simulink model "test_scan"  (Simulink 6.5)
settings: Solver=VariableStepDiscrete  StartTime=0.0  StopTime=5000  RelTol=1e-3
undefined symbols (not defined in the file or in its folder): sigbuilder_block
libraries: xbsIndex_r4 x78, nort_sysgenlib x8
settings Model: Creator=nort  LastModifiedBy=nort

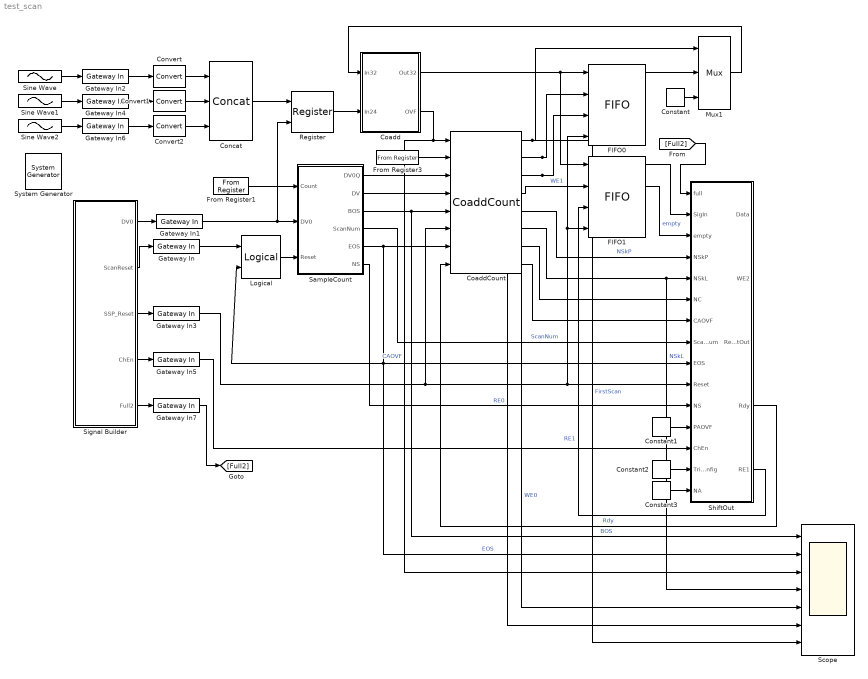
== system test_scan ==
  " System Generator" : xbsIndex_r4/ System Generator  Tag=genX  SystemSampleTime=-1  xilinxfamily=Virtex4  part=xc4vsx35  speed=-10  package=ff668  synthesis_tool=XST  directory=./netlist  testbench=off  simulink_period=1  sysclk_period=10  incr_netlist=off  trim_vbits=Everywhere in SubSystem  dbl_ovrd=According to Block Masks  core_generation=According to Block Masks  run_coregen=off  deprecated_control=off  eval_field=0  block_type=sysgen
      settings: block_version=9.2.01
  Coadd : Subsystem
  CoaddCount : nort_sysgenlib/CoaddCount  SystemSampleTime=-1
  Concat : xbsIndex_r4/Concat  num_inputs=3  dbl_ovrd=off  block_type=concat
      settings: block_version=9.2.01
  Constant : xbsIndex_r4/Constant  arith_type=Unsigned  const=0  n_bits=96  bin_pt=0  explicit_period=off  period=1  equ=P=C  opselect=C  inp2=PCIN>>17  opr=+  inp1=P  carry=CIN  dbl_ovrd=off  block_type=constant
      settings: block_version=9.2.01
  Constant1 : xbsIndex_r4/Constant  arith_type=Unsigned  const=0  n_bits=6  bin_pt=0  explicit_period=off  period=1  equ=P=C  opselect=C  inp2=PCIN>>17  opr=+  inp1=P  carry=CIN  dbl_ovrd=off  block_type=constant
      settings: block_version=9.2.01
  Constant2 : xbsIndex_r4/Constant  arith_type=Unsigned  const=0  n_bits=4  bin_pt=0  explicit_period=off  period=1  equ=P=C  opselect=C  inp2=PCIN>>17  opr=+  inp1=P  carry=CIN  dbl_ovrd=off  block_type=constant
      settings: block_version=9.2.01
  Constant3 : xbsIndex_r4/Constant  arith_type=Unsigned  const=1  n_bits=7  bin_pt=0  explicit_period=off  period=1  equ=P=C  opselect=C  inp2=PCIN>>17  opr=+  inp1=P  carry=CIN  dbl_ovrd=off  block_type=constant
      settings: block_version=9.2.01
  Convert : xbsIndex_r4/Convert  arith_type=Unsigned  n_bits=24  bin_pt=0  quantization=Truncate  overflow=Wrap  latency=0  dbl_ovrd=off  pipeline=off  block_type=convert
      settings: block_version=9.2.01
  Convert1 : xbsIndex_r4/Convert  arith_type=Unsigned  n_bits=24  bin_pt=0  quantization=Truncate  overflow=Wrap  latency=0  dbl_ovrd=off  pipeline=off  block_type=convert
      settings: block_version=9.2.01
  Convert2 : xbsIndex_r4/Convert  arith_type=Unsigned  n_bits=24  bin_pt=0  quantization=Truncate  overflow=Wrap  latency=0  dbl_ovrd=off  pipeline=off  block_type=convert
      settings: block_version=9.2.01
  FIFO0 : xbsIndex_r4/FIFO  depth=4K  percent_nbits=1  rst=on  en=off  use_dcount=off  use_almost_empty=off  almost_empty_thresh=2  use_almost_full=off  almost_full_thresh=14  dbl_ovrd=off  mem_type=Block RAM  block_type=fifo
      settings: block_version=9.2.01
  FIFO1 : xbsIndex_r4/FIFO  depth=4K  percent_nbits=1  rst=on  en=off  use_dcount=off  use_almost_empty=off  almost_empty_thresh=2  use_almost_full=off  almost_full_thresh=14  dbl_ovrd=off  mem_type=Block RAM  block_type=fifo
      settings: block_version=9.2.01
  From Register1 : xbsIndex_r4/From Register  shared_memory_name='NetSamples'  init=7  period=1  ownership=Locally owned and initialized  arith_type=Unsigned  n_bits=12  bin_pt=0  dbl_ovrd=off  block_type=fromreg
      settings: AttributesFormatString=From Register\n<< %<shared_memory_name> >>  infoedit="Register block that reads data to a shared memory register.  Delay of one sample period."  block_version=8.2
  From Register3 : xbsIndex_r4/From Register  shared_memory_name='NCoadd'  init=4  period=1  ownership=Locally owned and initialized  arith_type=Unsigned  n_bits=14  bin_pt=0  dbl_ovrd=off  block_type=fromreg
      settings: AttributesFormatString=<< %<shared_memory_name> >>  infoedit="Register block that reads data to a shared memory register.  Delay of one sample period."  block_version=9.2.01
  Gateway In : xbsIndex_r4/Gateway In  arith_type=Boolean  n_bits=16  bin_pt=14  quantization="Round  (unbiased: +/- Inf)"  overflow=Saturate  period=1  dbl_ovrd=off  timing_constraint=None  locs_specified=off  LOCs={}  block_type=gatewayin
      settings: infoedit="Gateway in block.  Converts inputs of type Simulink integer, double and fixed point to  Xilinx fixed point type.<P><P>Hardware notes:  In hardware these blocks become top level input ports."  block_version=9.2.01
  Gateway In1 : xbsIndex_r4/Gateway In  arith_type=Boolean  n_bits=16  bin_pt=14  quantization="Round  (unbiased: +/- Inf)"  overflow=Saturate  period=1  dbl_ovrd=off  timing_constraint=None  locs_specified=off  LOCs={}  block_type=gatewayin
      settings: infoedit="Gateway in block.  Converts inputs of type Simulink integer, double and fixed point to  Xilinx fixed point type.<P><P>Hardware notes:  In hardware these blocks become top level input ports."  block_version=9.2.01
  Gateway In2 : xbsIndex_r4/Gateway In  arith_type="Signed  (2's comp)"  n_bits=24  bin_pt=23  quantization="Round  (unbiased: +/- Inf)"  overflow=Saturate  period=1  dbl_ovrd=off  timing_constraint=None  locs_specified=off  LOCs={}  block_type=gatewayin
      settings: infoedit="Gateway in block.  Converts inputs of type Simulink integer, double and fixed point to  Xilinx fixed point type.<P><P>Hardware notes:  In hardware these blocks become top level input ports."  block_version=9.2.01
  Gateway In3 : xbsIndex_r4/Gateway In  arith_type=Boolean  n_bits=16  bin_pt=14  quantization="Round  (unbiased: +/- Inf)"  overflow=Saturate  period=1  dbl_ovrd=off  timing_constraint=None  locs_specified=off  LOCs={}  block_type=gatewayin
      settings: infoedit="Gateway in block.  Converts inputs of type Simulink integer, double and fixed point to  Xilinx fixed point type.<P><P>Hardware notes:  In hardware these blocks become top level input ports."  block_version=9.2.01
  Gateway In4 : xbsIndex_r4/Gateway In  arith_type="Signed  (2's comp)"  n_bits=24  bin_pt=0  quantization="Round  (unbiased: +/- Inf)"  overflow=Saturate  period=1  dbl_ovrd=off  timing_constraint=None  locs_specified=off  LOCs={}  block_type=gatewayin
      settings: infoedit="Gateway in block.  Converts inputs of type Simulink integer, double and fixed point to  Xilinx fixed point type.<P><P>Hardware notes:  In hardware these blocks become top level input ports."  block_version=9.2.01
  Gateway In5 : xbsIndex_r4/Gateway In  arith_type=Unsigned  n_bits=3  bin_pt=0  quantization="Round  (unbiased: +/- Inf)"  overflow=Saturate  period=1  dbl_ovrd=off  timing_constraint=None  locs_specified=off  LOCs={}  block_type=gatewayin
      settings: infoedit="Gateway in block.  Converts inputs of type Simulink integer, double and fixed point to  Xilinx fixed point type.<P><P>Hardware notes:  In hardware these blocks become top level input ports."  block_version=9.2.01
  Gateway In6 : xbsIndex_r4/Gateway In  arith_type="Signed  (2's comp)"  n_bits=24  bin_pt=0  quantization="Round  (unbiased: +/- Inf)"  overflow=Saturate  period=1  dbl_ovrd=off  timing_constraint=None  locs_specified=off  LOCs={}  block_type=gatewayin
      settings: infoedit="Gateway in block.  Converts inputs of type Simulink integer, double and fixed point to  Xilinx fixed point type.<P><P>Hardware notes:  In hardware these blocks become top level input ports."  block_version=9.2.01
  Gateway In7 : xbsIndex_r4/Gateway In  arith_type=Boolean  n_bits=1  bin_pt=0  quantization="Round  (unbiased: +/- Inf)"  overflow=Saturate  period=1  dbl_ovrd=off  timing_constraint=None  locs_specified=off  LOCs={}  block_type=gatewayin
      settings: infoedit="Gateway in block.  Converts inputs of type Simulink integer, double and fixed point to  Xilinx fixed point type.<P><P>Hardware notes:  In hardware these blocks become top level input ports."  block_version=9.2.01
  Logical : xbsIndex_r4/Logical  logical_function=OR  inputs=2  en=off  latency=0  precision=Full  arith_type=Unsigned  n_bits=16  bin_pt=0  align_bp=on  dbl_ovrd=off  block_type=logical
      settings: block_version=9.2.01
  Mux1 : xbsIndex_r4/Mux  inputs=2  en=off  latency=0  precision=Full  arith_type=Unsigned  n_bits=16  bin_pt=14  quantization=Truncate  overflow=Wrap  dbl_ovrd=off  block_type=mux
      settings: block_version=9.2.01
  Register : xbsIndex_r4/Register  init=0  rst=off  en=on  dbl_ovrd=off  block_type=register
      settings: block_version=9.2.01
  SampleCount : Subsystem
  Scope : Scope  NumInputPorts=7
      settings: TimeRange=5000  YMin=-0.25~-0.25~-0.25~-0.25~-0.25~-0.25~-0.25  YMax=1.25~1.25~1.25~1.25~1.25~1.25~1.25
  ShiftOut : Subsystem
  Signal Builder : Subsystem  Tag=STV Subsys  LoadFcn=sigbuilder_block('load');  StartFcn=sigbuilder_block('start');  StopFcn=sigbuilder_block('stop');  ClipboardFcn=sigbuilder_block('clipboard');  mask(Sigbuilder block){}
      mask help: Sigbuilder GUI
      mask init:
      | if ~strcmp(get_param(bdroot(gcbh),'SimulationStatus'),'stopped') tuvar = sigbuilder_block('maskInit'); end
      settings: CopyFcn=sigbuilder_block('copy');  DeleteFcn=sigbuilder_block('delete');  ModelCloseFcn=sigbuilder_block('modelClose');  PreSaveFcn=sigbuilder_block('preSave');  NameChangeFcn=sigbuilder_block('namechange');  OpenFcn=sigbuilder_block('open',[141.75 103.5 550.5 399.75 ]);  CloseFcn=sigbuilder_block('close');
      mask Display: plot(0,0,100,100,[10,10,40,40,10],[80,20,20,80,80],[40,10],[50,50], [40,27,10],[65,72,56],[40,25,25,10],[28,28,43,43]);
  Sine Wave : Sin  SampleTime=0
  Sine Wave1 : Sin  Phase=.3  SampleTime=0
  Sine Wave2 : Sin  Phase=.6  SampleTime=0
  wires:
  From Register1/1 -> SampleCount/1(Count)
  Constant3/1 -> ShiftOut/15(NA)
  Gateway In5/1 -> ShiftOut/13(ChEn)
  Gateway In1/1 -> Register/2, SampleCount/2(DV0)
  Coadd/1(Out32) -> FIFO0/1, FIFO1/1
  Register/1 -> Coadd/2(In24)
  Constant2/1 -> ShiftOut/14(TrigConfig)
  FIFO0/1 -> Mux1/2
  Constant/1 -> Mux1/3
  Mux1/1 -> Coadd/1(In32)
  Gateway In3/1 -> FIFO0/4, FIFO1/4, ShiftOut/10(Reset), CoaddCount/6
  SampleCount/5(EOS) -> Logical/2, Scope/2, ShiftOut/9(EOS), CoaddCount/7  "EOS"
  FIFO1/2 -> ShiftOut/3(empty)  "empty"
  SampleCount/3(BOS) -> CoaddCount/5, Scope/1  "BOS"
  From Register3/1 -> CoaddCount/2
  CoaddCount/1 -> Mux1/1, Scope/7  "FirstScan"
  SampleCount/2(DV) -> CoaddCount/4
  CoaddCount/2 -> FIFO0/2, Scope/5  "WE0"
  CoaddCount/4 -> FIFO1/2  "WE1"
  FIFO1/1 -> ShiftOut/2(SigIn)
  [Full2] -> ShiftOut/1(full)
  CoaddCount/5 -> ShiftOut/4(NSkP)  "NSkP"
  CoaddCount/6 -> Scope/4, ShiftOut/5(NSkL)  "NSkL"
  CoaddCount/7 -> ShiftOut/6(NC)
  SampleCount/4(ScanNum) -> ShiftOut/8(ScanNum)  "ScanNum"
  Constant1/1 -> ShiftOut/12(PAOVF)
  CoaddCount/8 -> ShiftOut/7(CAOVF)
  Coadd/2(OVF) -> CoaddCount/1, Scope/3  "CAOVF"
  SampleCount/6(NS) -> ShiftOut/11(NS)
  ShiftOut/5(RE1) -> FIFO1/3  "RE1"
  SampleCount/1(DV0Q) -> CoaddCount/3
  CoaddCount/3 -> FIFO0/3, Scope/6  "RE0"
  Concat/1 -> Register/1
  Gateway In2/1 -> Convert/1
  Gateway In4/1 -> Convert1/1
  Gateway In6/1 -> Convert2/1
  Sine Wave/1 -> Gateway In2/1
  Sine Wave1/1 -> Gateway In4/1
  Sine Wave2/1 -> Gateway In6/1
  Signal Builder/1(DV0) -> Gateway In1/1
  Signal Builder/2(ScanReset) -> Gateway In/1
  Signal Builder/3(SSP_Reset) -> Gateway In3/1
  Signal Builder/4(ChEn) -> Gateway In5/1
  Convert/1 -> Concat/1
  Convert1/1 -> Concat/2
  Convert2/1 -> Concat/3
  Logical/1 -> SampleCount/3(Reset)
  Gateway In/1 -> Logical/1
  Gateway In7/1 -> [Full2]
  Signal Builder/5(Full2) -> Gateway In7/1
  ShiftOut/4(Rdy) -> CoaddCount/8  "Rdy"

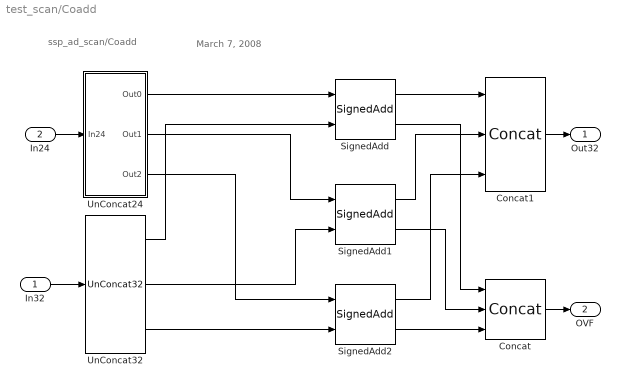
== system test_scan/Coadd ==
  note: ssp_ad_scan/Coadd
  note: March 7, 2008
  In32 : Inport
  In24 : Inport  Port=2
  Concat : xbsIndex_r4/Concat  num_inputs=3  dbl_ovrd=off  block_type=concat
      settings: block_version=9.2.01
  Concat1 : xbsIndex_r4/Concat  num_inputs=3  dbl_ovrd=off  block_type=concat
      settings: block_version=9.2.01
  SignedAdd : nort_sysgenlib/SignedAdd  SystemSampleTime=-1
  SignedAdd1 : nort_sysgenlib/SignedAdd  SystemSampleTime=-1
  SignedAdd2 : nort_sysgenlib/SignedAdd  SystemSampleTime=-1
  UnConcat24 : Subsystem
  UnConcat32 : nort_sysgenlib/UnConcat32  SystemSampleTime=-1
  Out32 : Outport
  OVF : Outport  Port=2
  wires:
  SignedAdd2/1 -> Concat1/3
  SignedAdd1/1 -> Concat1/2
  SignedAdd/1 -> Concat1/1
  UnConcat24/3(Out2) -> SignedAdd2/1
  UnConcat24/2(Out1) -> SignedAdd1/1
  UnConcat24/1(Out0) -> SignedAdd/1
  UnConcat32/1 -> SignedAdd/2
  Concat1/1 -> Out32/1
  UnConcat32/2 -> SignedAdd1/2
  UnConcat32/3 -> SignedAdd2/2
  In32/1 -> UnConcat32/1
  In24/1 -> UnConcat24/1(In24)
  Concat/1 -> OVF/1
  SignedAdd/2 -> Concat/1
  SignedAdd1/2 -> Concat/2
  SignedAdd2/2 -> Concat/3

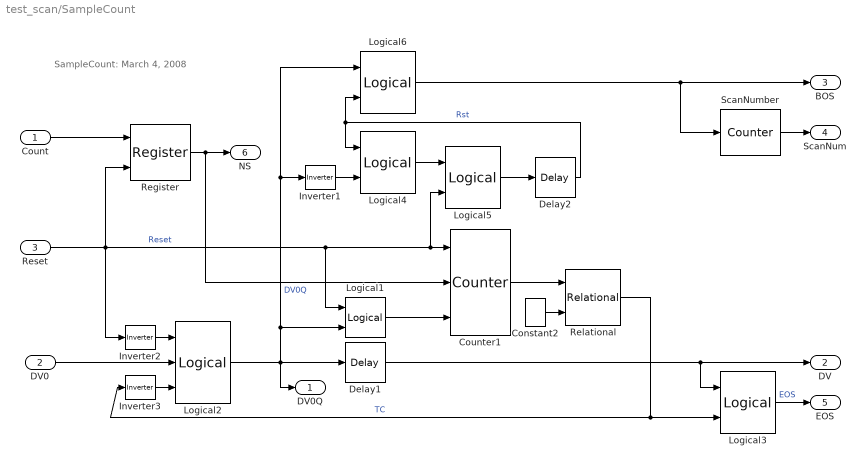
== system test_scan/SampleCount ==
  note: SampleCount: March 4, 2008
  Count : Inport
  DV0 : Inport  Port=2
  Reset : Inport  Port=3
  Constant2 : xbsIndex_r4/Constant  arith_type=Unsigned  const=0  n_bits=11  bin_pt=0  explicit_period=off  period=1  equ=P=C  opselect=C  inp2=PCIN>>17  opr=+  inp1=P  carry=CIN  dbl_ovrd=off  block_type=constant
      settings: block_version=8.2
  Counter1 : xbsIndex_r4/Counter  cnt_type=Free Running  cnt_to=Inf  operation=Down  start_count=0  cnt_by_val=1  arith_type=Unsigned  n_bits=12  bin_pt=0  load_pin=on  rst=off  en=on  explicit_period=off  period=1  dbl_ovrd=off  use_behavioral_HDL=off  use_rpm=off  block_type=counter
      settings: block_version=8.2
  Delay1 : xbsIndex_r4/Delay  en=off  latency=1  dbl_ovrd=off  reg_retiming=off  block_type=delay
      settings: block_version=9.2.01
  Delay2 : xbsIndex_r4/Delay  en=off  latency=1  dbl_ovrd=off  reg_retiming=off  block_type=delay
      settings: block_version=9.2.01
  Inverter1 : xbsIndex_r4/Inverter  en=off  latency=0  dbl_ovrd=off  block_type=inv
      settings: block_version=8.2
  Inverter2 : xbsIndex_r4/Inverter  en=off  latency=0  dbl_ovrd=off  block_type=inv
      settings: block_version=8.2
  Inverter3 : xbsIndex_r4/Inverter  en=off  latency=0  dbl_ovrd=off  block_type=inv
      settings: block_version=8.2
  Logical1 : xbsIndex_r4/Logical  logical_function=OR  inputs=2  en=off  latency=0  precision=Full  arith_type=Unsigned  n_bits=16  bin_pt=0  align_bp=on  dbl_ovrd=off  block_type=logical
      settings: block_version=8.2
  Logical2 : xbsIndex_r4/Logical  logical_function=AND  inputs=3  en=off  latency=0  precision=Full  arith_type=Unsigned  n_bits=1  bin_pt=0  align_bp=off  dbl_ovrd=off  block_type=logical
      settings: block_version=8.2
  Logical3 : xbsIndex_r4/Logical  logical_function=AND  inputs=2  en=off  latency=0  precision=Full  arith_type=Unsigned  n_bits=1  bin_pt=0  align_bp=off  dbl_ovrd=off  block_type=logical
      settings: block_version=8.2
  Logical4 : xbsIndex_r4/Logical  logical_function=AND  inputs=2  en=off  latency=0  precision=Full  arith_type=Unsigned  n_bits=1  bin_pt=0  align_bp=off  dbl_ovrd=off  block_type=logical
      settings: block_version=8.2
  Logical5 : xbsIndex_r4/Logical  logical_function=OR  inputs=2  en=off  latency=0  precision=Full  arith_type=Unsigned  n_bits=1  bin_pt=0  align_bp=off  dbl_ovrd=off  block_type=logical
      settings: block_version=8.2
  Logical6 : xbsIndex_r4/Logical  logical_function=AND  inputs=2  en=off  latency=0  precision=Full  arith_type=Unsigned  n_bits=1  bin_pt=0  align_bp=off  dbl_ovrd=off  block_type=logical
      settings: block_version=8.2
  Register : xbsIndex_r4/Register  init=0  rst=off  en=on  dbl_ovrd=off  block_type=register
      settings: block_version=9.2.01
  Relational : xbsIndex_r4/Relational  mode=a=b  en=off  latency=0  dbl_ovrd=off  block_type=relational
      settings: block_version=8.2
  ScanNumber : xbsIndex_r4/Counter  cnt_type=Free Running  cnt_to=Inf  operation=Up  start_count=0  cnt_by_val=1  arith_type=Unsigned  n_bits=32  bin_pt=0  load_pin=off  rst=off  en=on  explicit_period=off  period=1  dbl_ovrd=off  use_behavioral_HDL=off  use_rpm=off  block_type=counter
      settings: block_version=8.2
  DV0Q : Outport
  DV : Outport  Port=2
  BOS : Outport  Port=3
  ScanNum : Outport  Port=4
  EOS : Outport  Port=5
  NS : Outport  Port=6
  wires:
  Logical3/1 -> EOS/1  "EOS"
  Relational/1 -> Logical3/2, Inverter3/1  "TC"
  Reset/1 -> Logical1/1, Counter1/1, Logical5/2, Inverter2/1, Register/2  "Reset"
  Constant2/1 -> Relational/2
  Counter1/1 -> Relational/1
  ScanNumber/1 -> ScanNum/1
  Logical1/1 -> Counter1/3
  DV0/1 -> Logical2/2
  Inverter2/1 -> Logical2/1
  Inverter3/1 -> Logical2/3
  Logical2/1 -> Delay1/1, Logical1/2, Inverter1/1, Logical6/1, DV0Q/1  "DV0Q"
  Delay1/1 -> DV/1, Logical3/1
  Logical4/1 -> Logical5/1
  Inverter1/1 -> Logical4/2
  Logical5/1 -> Delay2/1
  Delay2/1 -> Logical4/1, Logical6/2  "Rst"
  Logical6/1 -> BOS/1, ScanNumber/1
  Count/1 -> Register/1
  Register/1 -> NS/1, Counter1/2

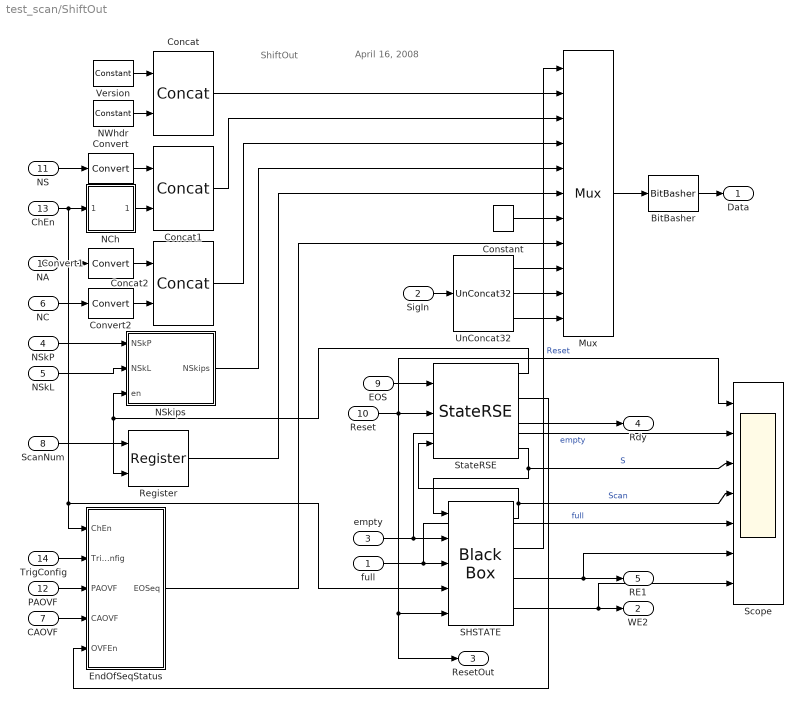
== system test_scan/ShiftOut ==
  note: ShiftOut
  note: April 16, 2008
  full : Inport
  SigIn : Inport  Port=2
  empty : Inport  Port=3
  NSkP : Inport  Port=4
  NSkL : Inport  Port=5
  NC : Inport  Port=6
  CAOVF : Inport  Port=7
  ScanNum : Inport  Port=8
  EOS : Inport  Port=9
  Reset : Inport  Port=10
  NS : Inport  Port=11
  PAOVF : Inport  Port=12
  ChEn : Inport  Port=13
  TrigConfig : Inport  Port=14
  NA : Inport  Port=15
  BitBasher : xbsIndex_r4/BitBasher  bitexpr=|  display_expr=off  sr_1=1  arith_type1=Unsigned  bin_pt1=0  sr_2=2  arith_type2=Unsigned  bin_pt2=0  sr_3=3  arith_type3=Unsigned  bin_pt3=0  sr_4=4  arith_type4=Unsigned  bin_pt4=0  dbl_ovrd=off  block_type=bitbasher
      | <html><head><meta name="qrichtext" content="1" /></head><body style="font-size:8pt;font-family:MS Shell Dlg">
      | <p>BE={LE[7:0],LE[15:8],LE[23:16],LE[31:24]}</p>
      | </body></html>
      settings: block_version=8.2
      settings: infoedit=|
      | Allows
      |      extraction, concatenation and augmentation of bits
  Concat : xbsIndex_r4/Concat  num_inputs=2  dbl_ovrd=off  block_type=concat
      settings: block_version=9.2.01
  Concat1 : xbsIndex_r4/Concat  num_inputs=2  dbl_ovrd=off  block_type=concat
      settings: block_version=9.2.01
  Concat2 : xbsIndex_r4/Concat  num_inputs=2  dbl_ovrd=off  block_type=concat
      settings: block_version=9.2.01
  Constant : xbsIndex_r4/Constant  arith_type=Unsigned  const=0  n_bits=32  bin_pt=0  explicit_period=off  period=1  equ=P=C  opselect=C  inp2=PCIN>>17  opr=+  inp1=P  carry=CIN  dbl_ovrd=off  block_type=constant
      settings: block_version=9.2.01
  Convert : xbsIndex_r4/Convert  arith_type=Unsigned  n_bits=16  bin_pt=0  quantization=Truncate  overflow=Wrap  latency=0  dbl_ovrd=off  pipeline=off  block_type=convert
      settings: block_version=9.2.01
  Convert1 : xbsIndex_r4/Convert  arith_type=Unsigned  n_bits=16  bin_pt=0  quantization=Truncate  overflow=Wrap  latency=0  dbl_ovrd=off  pipeline=off  block_type=convert
      settings: block_version=9.2.01
  Convert2 : xbsIndex_r4/Convert  arith_type=Unsigned  n_bits=16  bin_pt=0  quantization=Truncate  overflow=Wrap  latency=0  dbl_ovrd=off  pipeline=off  block_type=convert
      settings: block_version=9.2.01
  EndOfSeqStatus : Subsystem
  Mux : xbsIndex_r4/Mux  inputs=10  en=off  latency=0  precision=User Defined  arith_type="Signed  (2's comp)"  n_bits=32  bin_pt=0  quantization=Truncate  overflow=Saturate  dbl_ovrd=off  block_type=mux
      settings: block_version=8.2
  NCh : Subsystem
  NSkips : Subsystem
  NWhdr : xbsIndex_r4/Constant  arith_type=Unsigned  const=6  n_bits=16  bin_pt=0  explicit_period=off  period=1  equ=P=C  opselect=C  inp2=PCIN>>17  opr=+  inp1=P  carry=CIN  dbl_ovrd=off  block_type=constant
      settings: block_version=9.2.01
  Register : xbsIndex_r4/Register  init=0  rst=off  en=on  dbl_ovrd=off  block_type=register
      settings: block_version=9.2.01
  SHSTATE : xbsIndex_r4/Black Box  init_code=SHSTATE_config  sim_method=ISE Simulator  block_type=blackbox2
      settings: infoedit="Incorporates black box HDL and simulation model into a System Generator design.<P><P>You must supply a Black Box with certain information about the HDL component you would like to bring into System Generator. This information is provided through a Matlab function.<P><P>When \"Simulation mode\" is set to \"Inactive\", you will typically want to provide a separate simulation model by using a Simulation Multiplexer.<P>When \"Simulation mode\" is set to \"External co-simulator\", you must include a ModelSim block in the design."  block_version=9.2.01
  Scope : Scope  NumInputPorts=7
      settings: TickLabels=on  TimeRange=5000  YMin=-0.25~-0.25~-0.25~-0.25~-0.25~-0.25~-0.25  YMax=1.25~1.25~1.25~1.25~1.25~1.25~1.25
  StateRSE : nort_sysgenlib/StateRSE  SystemSampleTime=-1
  UnConcat32 : nort_sysgenlib/UnConcat32  SystemSampleTime=-1
  Version : xbsIndex_r4/Constant  arith_type=Unsigned  const=0  n_bits=16  bin_pt=0  explicit_period=off  period=1  equ=P=C  opselect=C  inp2=PCIN>>17  opr=+  inp1=P  carry=CIN  dbl_ovrd=off  block_type=constant
      settings: block_version=9.2.01
  Data : Outport
  WE2 : Outport  Port=2
  ResetOut : Outport  Port=3
  Rdy : Outport  Port=4
  RE1 : Outport  Port=5
  wires:
  Mux/1 -> BitBasher/1
  BitBasher/1 -> Data/1
  Reset/1 -> ResetOut/1, SHSTATE/5, StateRSE/2, Scope/1  "Reset"
  Version/1 -> Concat/1
  NWhdr/1 -> Concat/2
  Concat/1 -> Mux/2
  NS/1 -> Convert/1
  Convert/1 -> Concat1/1
  ChEn/1 -> NCh/1(ChEn), EndOfSeqStatus/1(ChEn), SHSTATE/4
  NCh/1(NCh) -> Concat1/2
  Concat1/1 -> Mux/3
  NA/1 -> Convert1/1
  NC/1 -> Convert2/1
  Concat2/1 -> Mux/4
  Convert1/1 -> Concat2/1
  Convert2/1 -> Concat2/2
  NSkips/1(NSkips) -> Mux/5
  NSkP/1 -> NSkips/1(NSkP)
  NSkL/1 -> NSkips/2(NSkL)
  ScanNum/1 -> Register/1
  Register/1 -> Mux/6
  Constant/1 -> Mux/7
  PAOVF/1 -> EndOfSeqStatus/3(PAOVF)
  CAOVF/1 -> EndOfSeqStatus/4(CAOVF)
  TrigConfig/1 -> EndOfSeqStatus/2(TrigConfig)
  EndOfSeqStatus/1(EOSeq) -> Mux/8
  UnConcat32/1 -> Mux/9
  UnConcat32/2 -> Mux/10
  UnConcat32/3 -> Mux/11
  SigIn/1 -> UnConcat32/1
  StateRSE/4 -> SHSTATE/1, Scope/3  "S"
  EOS/1 -> StateRSE/1
  empty/1 -> SHSTATE/2, Scope/2  "empty"
  full/1 -> SHSTATE/3, Scope/5  "full"
  StateRSE/2 -> EndOfSeqStatus/5(OVFEn)
  StateRSE/1 -> Register/2, NSkips/3(en)
  SHSTATE/4 -> WE2/1, Scope/7
  SHSTATE/3 -> RE1/1, Scope/6
  SHSTATE/2 -> Mux/1
  SHSTATE/1 -> StateRSE/3, Scope/4  "Scan"
  StateRSE/3 -> Rdy/1

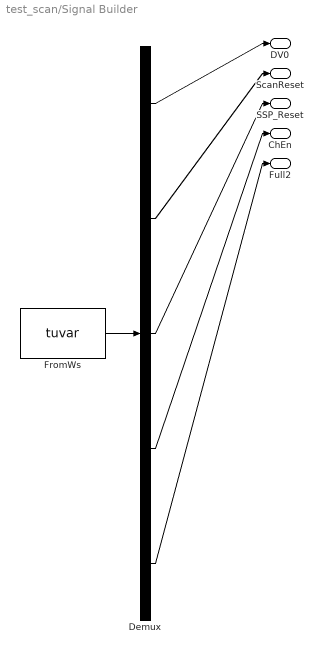
== system test_scan/Signal Builder ==
  Demux : Demux  Tag=STV Demux  Outputs=5
  FromWs : FromWorkspace  Tag=STV FromWs  VariableName=tuvar  SampleTime=0  SigBuilderData=DataTag1  VnvData=DataTag2
      SigBuilderData=|
      | channels(1).label = 'DV0'
      | channels(1).allXData = {[0 1 1 4 5 8 9 12 12 13 13 16 ... (4996 elements, 1x4996)], [0 1 1 4 5 8 9 12 12 13 13 16 ... (4996 elements, 1x4996)]}
      | channels(1).allYData = {[1 1 0 0 0 0 0 0 1 1 0 0 ... (4996 elements, 1x4996)], [1 1 0 0 0 0 0 0 1 1 0 0 ... (4996 elements, 1x4996)]}
      | channels(2).label = 'ScanReset'
      | channels(2).allXData = {[0 3 3 6 6 5000], [0 3 3 6 6 5000]}
      | channels(2).allYData = {[0 0 1 1 0 0], [0 0 1 1 0 0]}
      | channels(3).label = 'SSP_Reset'
      | channels(3).allXData = {[0 2 2 4 4 5000], [0 2 2 4 4 5000]}
      | channels(3).allYData = {[0 0 1 1 0 0], [0 0 1 1 0 0]}
      | channels(4).label = 'ChEn'
      | channels(4).allXData = {[0 5000], [0 5000]}
      | channels(4).allYData = {[4 4], [4 4]}
      | channels(5).label = 'Full2'
      | channels(5).allXData = {[0 230 230 500 500 539 539 1003 1003 1040 1040 1250 1250 5000], [0 230 500 539 539 1003 1003 1040 1040 1250 1250 5000]}
      | channels(5).allYData = {[0 0 1 1 0 0 1 1 0 0 1 1 0 0], [0 0 0 0 1 1 0 0 1 1 0 0]}
      | common.afterFinalStr = 'Extrapolate'
      | common.sampleTime = 0
      | dataSet(1).timeRange = [0 5000]
      | dataSet(1).name = 'Group 1'
      | dataSet(2).timeRange = [0 5000]
      | dataSet(2).name = 'Group 2'
  DV0 : Outport  Tag=STV Outport
  ScanReset : Outport  Tag=STV Outport  Port=2
  SSP_Reset : Outport  Tag=STV Outport  Port=3
  ChEn : Outport  Tag=STV Outport  Port=4
  Full2 : Outport  Tag=STV Outport  Port=5
  wires:
  FromWs/1 -> Demux/1
  Demux/1 -> DV0/1
  Demux/2 -> ScanReset/1
  Demux/3 -> SSP_Reset/1
  Demux/4 -> ChEn/1
  Demux/5 -> Full2/1

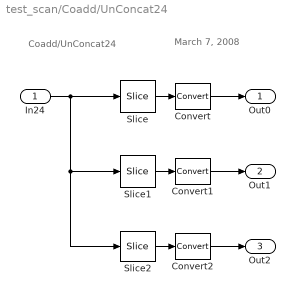
== system test_scan/Coadd/UnConcat24 ==
  note: Coadd/UnConcat24
  note: March 7, 2008
  In24 : Inport
  Convert : xbsIndex_r4/Convert  arith_type="Signed  (2's comp)"  n_bits=24  bin_pt=0  quantization=Truncate  overflow=Wrap  latency=0  dbl_ovrd=off  pipeline=off  block_type=convert
      settings: block_version=9.2.01
  Convert1 : xbsIndex_r4/Convert  arith_type="Signed  (2's comp)"  n_bits=24  bin_pt=0  quantization=Truncate  overflow=Wrap  latency=0  dbl_ovrd=off  pipeline=off  block_type=convert
      settings: block_version=9.2.01
  Convert2 : xbsIndex_r4/Convert  arith_type="Signed  (2's comp)"  n_bits=24  bin_pt=0  quantization=Truncate  overflow=Wrap  latency=0  dbl_ovrd=off  pipeline=off  block_type=convert
      settings: block_version=9.2.01
  Slice : xbsIndex_r4/Slice  nbits=24  boolean_output=off  mode=Lower Bit Location + Width  bit1=0  base1=MSB of Input  bit0=48  base0=LSB of Input  dbl_ovrd=off  block_type=slice
      settings: infoedit="Extracts a given range of bits from each input sample and presents it at the output.  The output type is ordinarily unsigned with binary point at zero, but can be Boolean when the slice is one bit wide.<P><P>Hardware notes: In hardware this block costs nothing."  block_version=9.2.01
  Slice1 : xbsIndex_r4/Slice  nbits=24  boolean_output=off  mode=Lower Bit Location + Width  bit1=0  base1=MSB of Input  bit0=24  base0=LSB of Input  dbl_ovrd=off  block_type=slice
      settings: infoedit="Extracts a given range of bits from each input sample and presents it at the output.  The output type is ordinarily unsigned with binary point at zero, but can be Boolean when the slice is one bit wide.<P><P>Hardware notes: In hardware this block costs nothing."  block_version=9.2.01
  Slice2 : xbsIndex_r4/Slice  nbits=24  boolean_output=off  mode=Lower Bit Location + Width  bit1=0  base1=MSB of Input  bit0=0  base0=LSB of Input  dbl_ovrd=off  block_type=slice
      settings: infoedit="Extracts a given range of bits from each input sample and presents it at the output.  The output type is ordinarily unsigned with binary point at zero, but can be Boolean when the slice is one bit wide.<P><P>Hardware notes: In hardware this block costs nothing."  block_version=9.2.01
  Out0 : Outport
  Out1 : Outport  Port=2
  Out2 : Outport  Port=3
  wires:
  In24/1 -> Slice2/1, Slice1/1, Slice/1
  Slice/1 -> Convert/1
  Slice1/1 -> Convert1/1
  Slice2/1 -> Convert2/1
  Convert/1 -> Out0/1
  Convert1/1 -> Out1/1
  Convert2/1 -> Out2/1

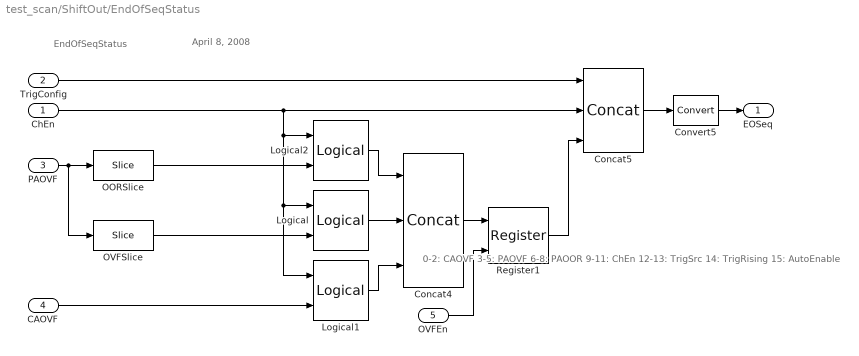
== system test_scan/ShiftOut/EndOfSeqStatus ==
  note: EndOfSeqStatus
  note: April 8, 2008
  note: 0-2: CAOVF
      | 3-5: PAOVF
      | 6-8: PAOOR
      | 9-11: ChEn
      | 12-13: TrigSrc
      | 14: TrigRising
      | 15: AutoEnable
  ChEn : Inport
  TrigConfig : Inport  Port=2
  PAOVF : Inport  Port=3
  CAOVF : Inport  Port=4
  OVFEn : Inport  Port=5
  Concat4 : xbsIndex_r4/Concat  num_inputs=3  dbl_ovrd=off  block_type=concat
      settings: block_version=9.2.01
  Concat5 : xbsIndex_r4/Concat  num_inputs=3  dbl_ovrd=off  block_type=concat
      settings: block_version=9.2.01
  Convert5 : xbsIndex_r4/Convert  arith_type=Unsigned  n_bits=32  bin_pt=0  quantization=Truncate  overflow=Wrap  latency=0  dbl_ovrd=off  pipeline=off  block_type=convert
      settings: block_version=9.2.01
  Logical : xbsIndex_r4/Logical  logical_function=AND  inputs=2  en=off  latency=0  precision=Full  arith_type=Unsigned  n_bits=16  bin_pt=0  align_bp=on  dbl_ovrd=off  block_type=logical
      settings: block_version=9.2.01
  Logical1 : xbsIndex_r4/Logical  logical_function=AND  inputs=2  en=off  latency=0  precision=Full  arith_type=Unsigned  n_bits=16  bin_pt=0  align_bp=on  dbl_ovrd=off  block_type=logical
      settings: block_version=9.2.01
  Logical2 : xbsIndex_r4/Logical  logical_function=AND  inputs=2  en=off  latency=0  precision=Full  arith_type=Unsigned  n_bits=16  bin_pt=0  align_bp=on  dbl_ovrd=off  block_type=logical
      settings: block_version=9.2.01
  OORSlice : xbsIndex_r4/Slice  nbits=3  boolean_output=off  mode=Lower Bit Location + Width  bit1=0  base1=MSB of Input  bit0=0  base0=LSB of Input  dbl_ovrd=off  block_type=slice
      settings: infoedit="Extracts a given range of bits from each input sample and presents it at the output.  The output type is ordinarily unsigned with binary point at zero, but can be Boolean when the slice is one bit wide.<P><P>Hardware notes: In hardware this block costs nothing."  block_version=9.2.01
  OVFSlice : xbsIndex_r4/Slice  nbits=3  boolean_output=off  mode=Lower Bit Location + Width  bit1=0  base1=MSB of Input  bit0=3  base0=LSB of Input  dbl_ovrd=off  block_type=slice
      settings: infoedit="Extracts a given range of bits from each input sample and presents it at the output.  The output type is ordinarily unsigned with binary point at zero, but can be Boolean when the slice is one bit wide.<P><P>Hardware notes: In hardware this block costs nothing."  block_version=9.2.01
  Register1 : xbsIndex_r4/Register  init=0  rst=off  en=on  dbl_ovrd=off  block_type=register
      settings: block_version=9.2.01
  EOSeq : Outport
  wires:
  Concat4/1 -> Register1/1
  Register1/1 -> Concat5/3
  Concat5/1 -> Convert5/1
  ChEn/1 -> Logical/1, Logical1/1, Logical2/1, Concat5/2
  TrigConfig/1 -> Concat5/1
  Convert5/1 -> EOSeq/1
  OVFEn/1 -> Register1/2
  Logical/1 -> Concat4/2
  CAOVF/1 -> Logical1/2
  Logical1/1 -> Concat4/3
  PAOVF/1 -> OORSlice/1, OVFSlice/1
  OORSlice/1 -> Logical2/2
  OVFSlice/1 -> Logical/2
  Logical2/1 -> Concat4/1

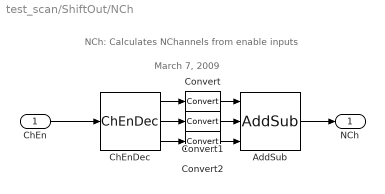
== system test_scan/ShiftOut/NCh ==
  note: NCh: Calculates NChannels from enable inputs
  note: March 7, 2009
  ChEn : Inport
  AddSub : xbsIndex_r4/AddSub  mode=Addition  use_carryin=on  use_carryout=off  en=off  latency=0  precision=User Defined  arith_type=Unsigned  n_bits=16  bin_pt=0  quantization=Truncate  overflow=Wrap  dbl_ovrd=off  use_behavioral_HDL=off  pipelined=off  use_rpm=on  block_type=addsub
      settings: block_version=9.2.01
  ChEnDec : nort_sysgenlib/ChEnDec  SystemSampleTime=-1
  Convert : xbsIndex_r4/Convert  arith_type=Unsigned  n_bits=1  bin_pt=0  quantization=Truncate  overflow=Wrap  latency=0  dbl_ovrd=off  pipeline=off  block_type=convert
      settings: block_version=9.2.01
  Convert1 : xbsIndex_r4/Convert  arith_type=Unsigned  n_bits=1  bin_pt=0  quantization=Truncate  overflow=Wrap  latency=0  dbl_ovrd=off  pipeline=off  block_type=convert
      settings: block_version=9.2.01
  Convert2 : xbsIndex_r4/Convert  arith_type=Unsigned  n_bits=1  bin_pt=0  quantization=Truncate  overflow=Wrap  latency=0  dbl_ovrd=off  pipeline=off  block_type=convert
      settings: block_version=9.2.01
  NCh : Outport
  wires:
  AddSub/1 -> NCh/1
  ChEn/1 -> ChEnDec/1
  ChEnDec/1 -> Convert/1
  ChEnDec/2 -> Convert1/1
  ChEnDec/3 -> Convert2/1
  Convert/1 -> AddSub/1
  Convert1/1 -> AddSub/2
  Convert2/1 -> AddSub/3

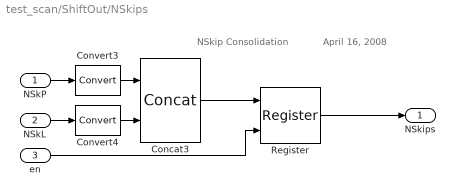
== system test_scan/ShiftOut/NSkips ==
  note: NSkip Consolidation
  note: April 16, 2008
  NSkP : Inport
  NSkL : Inport  Port=2
  en : Inport  Port=3
  Concat3 : xbsIndex_r4/Concat  num_inputs=2  dbl_ovrd=off  block_type=concat
      settings: block_version=9.2.01
  Convert3 : xbsIndex_r4/Convert  arith_type=Unsigned  n_bits=16  bin_pt=0  quantization=Truncate  overflow=Wrap  latency=0  dbl_ovrd=off  pipeline=off  block_type=convert
      settings: block_version=9.2.01
  Convert4 : xbsIndex_r4/Convert  arith_type=Unsigned  n_bits=16  bin_pt=0  quantization=Truncate  overflow=Wrap  latency=0  dbl_ovrd=off  pipeline=off  block_type=convert
      settings: block_version=9.2.01
  Register : xbsIndex_r4/Register  init=0  rst=off  en=on  dbl_ovrd=off  block_type=register
      settings: block_version=9.2.01
  NSkips : Outport
  wires:
  Convert3/1 -> Concat3/1
  Convert4/1 -> Concat3/2
  NSkP/1 -> Convert3/1
  NSkL/1 -> Convert4/1
  Concat3/1 -> Register/1
  Register/1 -> NSkips/1
  en/1 -> Register/2
